simulink model "FOC_BANG"  (R2022b)
settings: Solver=VariableStepAuto  StartTime=0.0  StopTime=12  RelTol=1e-3
InitFcn:
  | FOC_BANG
values from neighbouring files (symbols this model uses):
  eps_i = k_eps*Is_n*sqrt(2)    [FOC_BANG_Script.m]
  f_n = 300    [FOC_BANG_Script.m]    (also in IFOCdatav6.m)
  Im_n = k_im*Is_n    [FOC_BANG_Script.m]    (also in IFOCdatav6.m)
  J = 5    [Data.m]    (also in FOC_BANG_Script.m; IFOCdatav6.m)
  ki_w = 0.5*(kp_w^2)/J    (= 3.92607044657)    [FOC_BANG_Script.m]    (also in IFOCdatav6.m = 613.448507277)
  kp_w = T_n/(0.05*wr_n)/5    (= 6.2658362942)    [FOC_BANG_Script.m]    (also in IFOCdatav6.m = 78.3229536775)
  Lm = Phi_n/Im_n    [FOC_BANG_Script.m]    (also in IFOCdatav6.m)
  Lr = Ltot/2    [FOC_BANG_Script.m]    (also in IFOCdatav6.m)
  Ls = Ltot/2    [FOC_BANG_Script.m]    (also in IFOCdatav6.m)
  p = 6    [Data.m]    (also in FOC_BANG_Script.m; IFOCdatav6.m)
  P_n = 150000    [FOC_BANG_Script.m]    (also in IFOCdatav6.m)
  Rr = Rs    [FOC_BANG_Script.m]    (also in IFOCdatav6.m)
  Rs = (Pjs/3)/(Is_n^2)    [FOC_BANG_Script.m]    (also in IFOCdatav6.m)
  sigma_r = Lr/Lm    [FOC_BANG_Script.m]    (also in IFOCdatav6.m)
  T_n = P_n/wr_n    (= 484.735867285)    [FOC_BANG_Script.m]    (also in IFOCdatav6.m)
  T_rate_max = T_n/0.01    (= 48473.5867285)    [FOC_BANG_Script.m]    (also in IFOCdatav6.m)
  Tk_n = k_lim*T_n    (= 969.47173457)    [FOC_BANG_Script.m]    (also in IFOCdatav6.m = 1211.83966821)
  Tr = Lm*(1+sigma_r)/Rr    [FOC_BANG_Script.m]    (also in IFOCdatav6.m)
  Ts = 1/fs    (= 5e-05)    [FOC_BANG_Script.m]    (also in IFOCdatav6.m = 0.0001)
  Vdc = 350    [Data.m]    (also in FOC_BANG_Script.m; IFOCdatav6.m)
  Vs_n = 220    [FOC_BANG_Script.m]    (also in IFOCdatav6.m)
  wr_n = w_n/p*(1-s_n)    (= 309.446876379)    [FOC_BANG_Script.m]    (also in IFOCdatav6.m)
undefined symbols (not defined in the file or in its folder): sigbuilder_block
libraries: spsControlledVoltageSourceLib x3, spsCurrentMeasurementLib x3, spsAsynchronousMachineSIUnitsLib x1, spsGroundLib x1, slpidlib x1, sps_lib x1
settings Model: Creator=39388  LastModifiedBy=v4pal
settings SolverCC: AlgebraicLoopSolver=TrustRegion
settings DebuggingCC: UnconnectedInputMsg=warning  UnconnectedOutputMsg=warning  UnconnectedLineMsg=warning  SFMachineParentedDataDiag=warning
settings ModelReferenceCC: EnableRefExpFcnMdlSchedulingChecks=on
settings RTWCC: DLArmComputeVersion=19.05

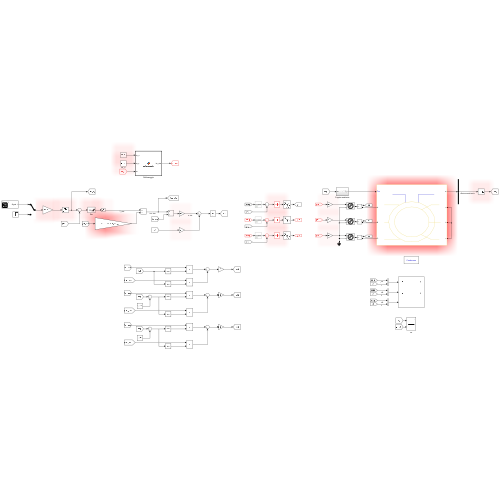
[thumbnail: Simulink's stored preview of the top-level diagram]
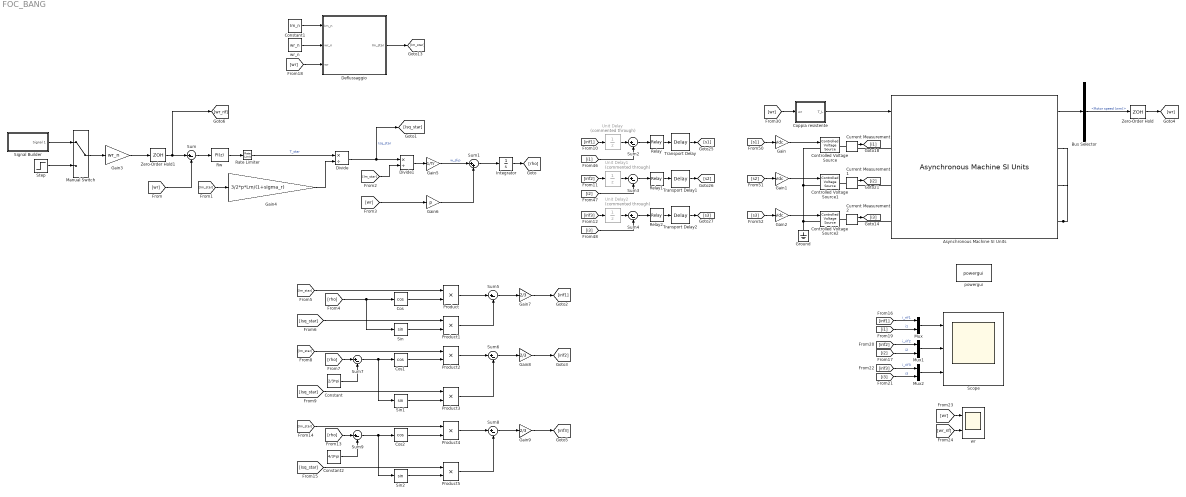
== system FOC_BANG ==
  Asynchronous Machine SI Units : spsAsynchronousMachineSIUnitsLib/Asynchronous Machine SI Units  RotorType=Wound  PresetModel=No  MechanicalLoad=Torque Tm  ShowDetailedParameters=on  ReferenceFrame=Rotor  Units=SI  MeasurementBus=off  NominalParameters=[P_n Vs_n f_n]  VoltageRatio=1  Stator=[Rs Ls]  Rotor=[Rr Lr]  Cage1=[0.4155 0.002066]  Cage2=[0.4168 0.0003495]  Lm=Lm  Mechanical=[J 0 p/2]  PolePairs=2  InitialConditions=[1 0 0 0 0 0 0 0]  SimulateSaturation=off  Saturation=[14.03593122, 27.81365428, 53.79336849, 72.68890987, 97.98006896, 148.6815601, 215.7428561, 302.9841135, 428.7778367 ; 230, 322, 414, 460, 506, 552, 598, 644, 690]  LoadFlowParameters=1492000  TsPowergui=0  TsBlock=-1  IterativeModel=Trapezoidal non iterative  IterativeDiscreteModel=Trapezoidal non iterative  Pmec=1.492e+006
  Bus Selector : BusSelector  OutputSignals=Mechanical.Rotor speed (wm)
  Constant : Constant  Value=2/3*pi
  Constant1 : Constant  Value=Im_n
  Constant2 : Constant  Value=4/3*pi
  Controlled Voltage Source : spsControlledVoltageSourceLib/Controlled Voltage Source  Initialize=on  Source_Type=AC  Amplitude=0  Phase=0  Frequency=0  Measurements=None
  Controlled Voltage Source1 : spsControlledVoltageSourceLib/Controlled Voltage Source  Initialize=on  Source_Type=AC  Amplitude=0  Phase=0  Frequency=0  Measurements=None
  Controlled Voltage Source2 : spsControlledVoltageSourceLib/Controlled Voltage Source  Initialize=on  Source_Type=AC  Amplitude=0  Phase=0  Frequency=0  Measurements=None
  Coppia resistente : Subsystem
  Cos : Trigonometry  Operator=cos
  Cos1 : Trigonometry  Operator=cos
  Cos2 : Trigonometry  Operator=cos
  Current Measurement : spsCurrentMeasurementLib/Current Measurement  PhasorSimulation=off  OutputType=Complex  PSBequivalent=0
  Current Measurement1 : spsCurrentMeasurementLib/Current Measurement  PhasorSimulation=off  OutputType=Complex  PSBequivalent=0
  Current Measurement2 : spsCurrentMeasurementLib/Current Measurement  PhasorSimulation=off  OutputType=Complex  PSBequivalent=0
  Deflussaggio : MATLAB Function  TreatAsAtomicUnit=on
  Divide : Product  Inputs=*/
  Divide1 : Product  Inputs=*/
  Gain : Gain  Gain=Vdc
  Gain1 : Gain  Gain=Vdc
  Gain2 : Gain  Gain=Vdc
  Gain3 : Gain  Gain=wr_n
  Gain4 : Gain  Gain=3/2*p*Lm/(1+sigma_r)
  Gain5 : Gain  Gain=1/Tr
  Gain6 : Gain  Gain=p
  Gain7 : Gain  Gain=2/3
  Gain8 : Gain  Gain=2/3
  Gain9 : Gain  Gain=2/3
  Ground : spsGroundLib/Ground  LConnTagsString=a
  Integrator : Integrator
  Manual Switch : ManualSwitch
  Mux : Mux  Inputs=2
  Mux1 : Mux  Inputs=2
  Mux2 : Mux  Inputs=2
  Product{,1..5} (6 alike) : Product
  Rate Limiter : RateLimiter  RisingSlewLimit=T_rate_max  FallingSlewLimit=-T_rate_max  SampleTimeMode=inherited
  Relay : Relay  OnSwitchValue=eps_i  OffSwitchValue=-eps_i
  Relay1 : Relay  OnSwitchValue=eps_i  OffSwitchValue=-eps_i
  Relay2 : Relay  OnSwitchValue=eps_i  OffSwitchValue=-eps_i
  Rw : slpidlib/PID Controller  Controller=PI  Form=Parallel  TimeDomain=Discrete-time  UseExternalTs=off  SampleTime=Ts  IntegratorMethod=Trapezoidal  FilterMethod=Forward Euler  ControllerParametersSource=internal  P=kp_w  I=ki_w  UseKiTs=off  D=0  N=100  UseFilter=on  TunerSelectOption=Frequency Response Based  InitialConditionSource=internal  InitialConditionForIntegrator=0  InitialConditionForFilter=0  DifferentiatorICPrevScaledInput=0  ExternalReset=none  TrackingMode=off  Kt=1  LimitOutput=on  SatLimitsSource=internal  UpperSaturationLimit=Tk_n  LowerSaturationLimit=-Tk_n  LinearizeAsGain=on  AntiWindupMode=clamping  Kb=1  LimitIntegrator=off  UpperIntegratorSaturationLimit=inf  LowerIntegratorSaturationLimit=-inf  POutMin=[]  POutMax=[]  IOutMin=[]  IOutMax=[]  DOutMin=[]  DOutMax=[]  NOutMin=[]  NOutMax=[]  SumOutMin=[]  SumOutMax=[]  SaturationOutMin=[]  SaturationOutMax=[]  PParamMin=[]  PParamMax=[]  IParamMin=[]  IParamMax=[]  DParamMin=[]  DParamMax=[]  NParamMin=[]  NParamMax=[]  KbParamMin=[]  KbParamMax=[]  KtParamMin=[]  KtParamMax=[]  KbOutMin=[]  KbOutMax=[]  KtOutMin=[]  KtOutMax=[]  IntegratorOutMin=[]  IntegratorOutMax=[]  FilterOutMin=[]  FilterOutMax=[]  SumI1OutMin=[]  SumI1OutMax=[]  SumI2OutMin=[]  SumI2OutMax=[]  SumI3OutMin=[]  SumI3OutMax=[]  SumI4OutMin=[]  SumI4OutMax=[]  SumDOutMin=[]  SumDOutMax=[]  DifferentiatorOutMin=[]  DifferentiatorOutMax=[]  FilterDiffOutCoefMin=[]  FilterDiffOutCoefMax=[]  ReciprocalOutMin=[]  ReciprocalOutMax=[]  SumDenOutMin=[]  SumDenOutMax=[]  SumNumOutMin=[]  SumNumOutMax=[]  DivideOutMin=[]  DivideOutMax=[]  UdiffTsProdOutMin=[]  UdiffTsProdOutMax=[]  NTsProdOutMin=[]  NTsProdOutMax=[]  UintegralTsProdOutMin=[]  UintegralTsProdOutMax=[]  UngainTsProdOutMin=[]  UngainTsProdOutMax=[]  ClampingZeroOutDataTypeStr=Inherit: Inherit via back propagation  ClampingZeroOutMin=[]  ClampingZeroOutMax=[]  FilterDenConstantOutDataTypeStr=Inherit: Inherit via back propagation  FilterDenConstantOutMin=[]  FilterDenConstantOutMax=[]  PCopyOutDataTypeStr=Inherit: Inherit via back propagation  PCopyOutMin=[]  PCopyOutMax=[]  NCopyOutDataTypeStr=Inherit: Inherit via back propagation  NCopyOutMin=[]  NCopyOutMax=[]  IntegratorContinuousStateAttributes=''  IntegratorStateMustResolveToSignalObject=off  IntegratorRTWStateStorageClass=Auto  FilterContinuousStateAttributes=''  FilterStateMustResolveToSignalObject=off  FilterRTWStateStorageClass=Auto  ParallelPVariant=InternalParameters  IdealPVariant=Disabled  IVariant=InternalParameters  DVariant=Disabled  IntegratorVariant=Discrete  SatVariant=Enabled  AWVariant=DiscClampingParallel  PCopyVariant=Disabled  TRVariant=Disabled  FdbkBlocksVariant=Feedback  IdealPFdbkVariant=Passthrough  SatFdbkVariant=Passthrough  DerivativeFilterVariant=Disabled  NVariant=Disabled  NCopyVariant=Disabled_SignalSpec  FilterICVariant=Disabled  IntegratorICVariant=InternalICs  ExternalResetVariant=Disabled  TRSumVariant=Passthrough  SumFdbkVariant=Enabled  SumVariant=Sum_PI  TsampFilterVariant=InternalTs  TsampNgainVariant=Passthrough  TsampIntegralVariant=Passthrough  ExternalSaturationOutDataTypeStr=Inherit: Same as second input
  Scope : Scope  NumInputPorts=3
  Signal Builder : Subsystem  Tag=STV Subsys  LoadFcn=sigbuilder_block('load');  StartFcn=sigbuilder_block('start');  StopFcn=sigbuilder_block('stop');  ClipboardFcn=sigbuilder_block('clipboard');  mask(Sigbuilder block){tuvar=[0:10]}
      mask help: Simulink:masks:SigbuilderBlock_MD
      mask init:
      | if ~strcmp(get_param(bdroot(gcbh),'SimulationStatus'),'stopped') tuvar = sigbuilder_block('maskInit'); end
      settings: CopyFcn=sigbuilder_block('copy');  DeleteFcn=sigbuilder_block('delete');  ModelCloseFcn=sigbuilder_block('modelClose');  PreSaveFcn=sigbuilder_block('preSave');  PauseFcn=sigbuilder_block('pause');  ContinueFcn=sigbuilder_block('continue');  NameChangeFcn=sigbuilder_block('namechange');  OpenFcn=sigbuilder_block('open',[437.6 199.2 550.4 400 ]);  CloseFcn=sigbuilder_block('close');
      mask Display: plot(0, 0, 100, 100,[2, 2, 32, 32, 2], [68, 8, 8, 68, 68],[32, 2], [38, 38], [32, 19, 2],[53, 60, 44], [32, 17, 17, 2],[16, 16, 31, 31]);txt = getActiveGroup(gcbh);text(2, 100, txt,'verticalAlignment', 'top');
  Sin : Trigonometry
  Sin1 : Trigonometry
  Sin2 : Trigonometry
  Step : Step  Time=0.2  SampleTime=0
  Sum{,2..9} (9 alike) : Sum  Inputs=|+-
  Sum1 : Sum  Inputs=|++
  Transport Delay : TransportDelay  DelayTime=1e-6
  Transport Delay1 : TransportDelay  DelayTime=1e-6
  Transport Delay2 : TransportDelay  DelayTime=1e-6
  Unit Delay : UnitDelay  Commented=through  SampleTime=Ts  HasFrameUpgradeWarning=on
  Unit Delay1 : UnitDelay  Commented=through  SampleTime=Ts  HasFrameUpgradeWarning=on
  Unit Delay2 : UnitDelay  Commented=through  SampleTime=Ts  HasFrameUpgradeWarning=on
  Zero-Order Hold : ZeroOrderHold  SampleTime=Ts
  Zero-Order Hold1 : ZeroOrderHold  SampleTime=Ts
  powergui : sps_lib/powergui  Priority=1  SimulationMode=Continuous  SampleTime=50e-6  frequency=60  Iterations=50  frequencyindice=0  Pbase=100e6  ErrMax=1e-4  UnitsV=kV  UnitsW=MW  buscounter=0  FunctionMessages=off  echomessages=off  EnableUseOfTLC=off  CurrentSourceSwitches=off  DisableSnubberDevices=off  DisableRonSwitches=off  DisableVfSwitches=off  DisplayEquations=off  AutomaticDiscreteSolvers=off  SolverType=Tustin/Backward Euler (TBE)  Interpol=off  ExternalGateDelay=off  methode=off  Ts=100  x0status=blocks  SPID=on  SwTol=0  HookPort=off  NonlinearTolerance=1e-4  nMaxIteration=100  ContinueOnMaxIteration=off  RestoreLinks=warning  ResistiveCurrentMeasurement=off  Frange=[0:2:500]  Ylog=off  Xlog=on  ShowGrid=off  save=off  variable=ZData  structure=0  ZoomFFT=off  StartTime=0.0  cycles=1  DisplayStyle=1  fundamental=60  FreqAxis=off  MaxFrequency=1000  frequencyindicesteady=1  RmsSteady=1  display=off
  wr : Scope  NumInputPorts=2
  wr_n : Constant  Value=wr_n
  wires:
  Asynchronous Machine SI Units/1 -> Bus Selector/1
  Current Measurement1/1 -> [i2]
  Bus Selector/1 -> Zero-Order Hold/1  "<Rotor speed (wm)>"
  Current Measurement2/1 -> [i3]
  [wr] -> Coppia resistente/1(wr)
  Coppia resistente/1(T_L) -> Asynchronous Machine SI Units/1
  Gain2/1 -> Controlled Voltage Source2/1
  Gain1/1 -> Controlled Voltage Source1/1
  [s2] -> Gain1/1
  [s3] -> Gain2/1
  Current Measurement/1 -> [i1]
  Gain/1 -> Controlled Voltage Source/1
  [s1] -> Gain/1
  Zero-Order Hold/1 -> [wr]
  [irif2] -> Unit Delay1/1
  [irif1] -> Unit Delay/1
  Transport Delay/1 -> [s1]
  Transport Delay2/1 -> [s3]
  Unit Delay/1 -> Sum2/1
  Sum4/1 -> Relay2/1
  Unit Delay2/1 -> Sum4/1
  [irif3] -> Unit Delay2/1
  Transport Delay1/1 -> [s2]
  Unit Delay1/1 -> Sum3/1
  [i3] -> Sum4/2
  Relay/1 -> Transport Delay/1
  [i1] -> Sum2/2
  Relay1/1 -> Transport Delay1/1
  Sum2/1 -> Relay/1
  [i2] -> Sum3/2
  Relay2/1 -> Transport Delay2/1
  Sum3/1 -> Relay1/1
  Deflussaggio/1(Im_star) -> [Im_star]
  Constant1/1 -> Deflussaggio/1(Im_n)
  [wr] -> Deflussaggio/3(wr)
  wr_n/1 -> Deflussaggio/2(wr_n)
  [wr] -> Sum/2
  Sum/1 -> Rw/1
  Zero-Order Hold1/1 -> [wr_rif], Sum/1
  Gain3/1 -> Zero-Order Hold1/1
  Rw/1 -> Rate Limiter/1
  [Im_star] -> Gain4/1
  Rate Limiter/1 -> Divide/1  "T_star"
  Gain4/1 -> Divide/2
  Divide/1 -> [Isq_star], Divide1/1  "Isq_star"
  [Im_star] -> Divide1/2
  Divide1/1 -> Gain5/1
  Gain5/1 -> Sum1/1  "w_slip"
  Gain6/1 -> Sum1/2
  Sum1/1 -> Integrator/1
  [wr] -> Gain6/1
  Integrator/1 -> [rho]
  Sum5/1 -> Gain7/1
  Sin/1 -> Product1/2
  Cos/1 -> Product/2
  Product/1 -> Sum5/1
  Product1/1 -> Sum5/2
  [Im_star] -> Product/1
  [Isq_star] -> Product1/1
  [rho] -> Cos/1, Sin/1
  Gain7/1 -> [irif1]
  Sin1/1 -> Product3/2
  [Isq_star] -> Product3/1
  Sum6/1 -> Gain8/1
  Product3/1 -> Sum6/2
  Cos1/1 -> Product2/2
  Product2/1 -> Sum6/1
  Gain8/1 -> [irif2]
  [Im_star] -> Product2/1
  [rho] -> Sum7/1
  Sum7/1 -> Sin1/1, Cos1/1
  Constant/1 -> Sum7/2
  Sin2/1 -> Product5/2
  [Im_star] -> Product4/1
  Gain9/1 -> [irif3]
  Product5/1 -> Sum8/2
  Cos2/1 -> Product4/2
  Sum8/1 -> Gain9/1
  [Isq_star] -> Product5/1
  [rho] -> Sum9/1
  Product4/1 -> Sum8/1
  Constant2/1 -> Sum9/2
  Sum9/1 -> Sin2/1, Cos2/1
  Manual Switch/1 -> Gain3/1
  Signal Builder/1(Signal 1) -> Manual Switch/1
  Step/1 -> Manual Switch/2
  [i1] -> Mux/2  "i1"
  [i2] -> Mux1/2  "i2"
  Mux/1 -> Scope/1
  Mux1/1 -> Scope/2
  [irif1] -> Mux/1  "i_rif1"
  [irif2] -> Mux1/1  "i_rif2"
  [irif3] -> Mux2/1  "i_rif3"
  [i3] -> Mux2/2  "i3"
  Mux2/1 -> Scope/3
  [wr_rif] -> wr/2
  [wr] -> wr/1
  connections:
  Asynchronous Machine SI Units/RConn3 -- Asynchronous Machine SI Units/RConn1 -- Asynchronous Machine SI Units/RConn2
  Controlled Voltage Source/LConn1 -- Ground/LConn1 -- Controlled Voltage Source2/LConn1 -- Controlled Voltage Source1/LConn1
  Asynchronous Machine SI Units/LConn3 -- Current Measurement2/RConn1
  Asynchronous Machine SI Units/LConn1 -- Current Measurement/RConn1
  Controlled Voltage Source1/RConn1 -- Current Measurement1/LConn1
  Asynchronous Machine SI Units/LConn2 -- Current Measurement1/RConn1
  Controlled Voltage Source2/RConn1 -- Current Measurement2/LConn1
  Current Measurement/LConn1 -- Controlled Voltage Source/RConn1

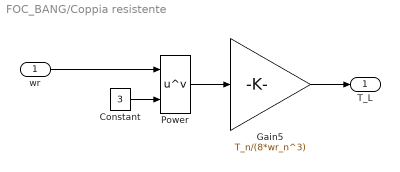
== system FOC_BANG/Coppia resistente ==
  wr : Inport
  Constant : Constant  Value=3
  Gain5 : Gain  Gain=T_n/(8*wr_n^3)
  Power : Math  Operator=pow
  T_L : Outport
  wires:
  Power/1 -> Gain5/1
  Constant/1 -> Power/2
  Gain5/1 -> T_L/1
  wr/1 -> Power/1

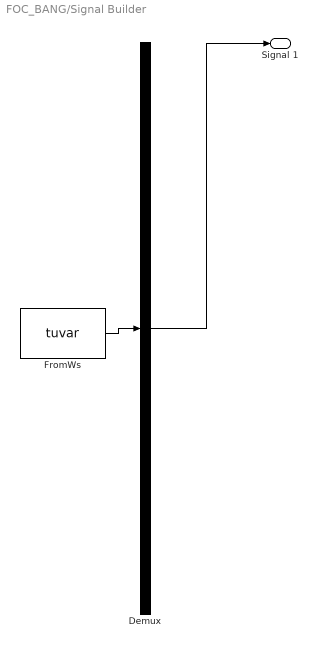
== system FOC_BANG/Signal Builder ==
  Demux : Demux  Tag=STV Demux  Outputs=1
      settings: DisplayOption=none
  FromWs : FromWorkspace  Tag=STV FromWs  VariableName=tuvar
      SigBuilderData=|
      | common.afterFinalStr = 'Extrapolate'
      | common.sampleTime = 0
      | dataSet.timeRange = [0 12]
      | dataSet.name = 'Group 1'
      | sbobj.Groups.Name = 'Group 1'
      | sbobj.Groups.Signals.Name = 'Signal 1'
      | sbobj.Groups.Signals.XData = [0 0.2 0.2 6 6 12]
      | sbobj.Groups.Signals.YData = [0 0 1 1 2 2]
      | sbobj.Groups.TimeRange = [0 12]
  Signal 1 : Outport  Tag=STV Outport
  wires:
  Demux/1 -> Signal 1/1
  FromWs/1 -> Demux/1

== matlab function FOC_BANG/Deflussaggio ==
  data: Im_n input; Im_star output; wr_n input; wr input
function Im_star = deflussaggio(Im_n,wr_n,wr)
k = Im_n*wr_n;

if wr > wr_n
    Im_star = k/wr;
else if wr < -wr_n
    Im_star = -k/wr;
    else
    Im_star = Im_n;
end
end
end
